simulink model "pid"  (R2018a)
settings: Solver=VariableStepAuto  StartTime=0.0  StopTime=10.0  RelTol=1e-3
settings Model: Creator=hp  LastModifiedBy=hp

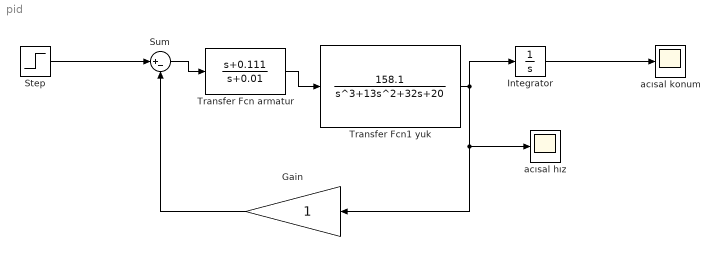
== system pid ==
  Gain : Gain
  Integrator : Integrator
  Step : Step  SampleTime=0
  Sum : Sum  Inputs=|+-
  Transfer Fcn armatur : TransferFcn  Numerator=[1 0.111]  Denominator=[1 0.01]
  Transfer Fcn1 yuk : TransferFcn  Numerator=[158.1]  Denominator=[1 13 32 20]
  acısal hız : Scope
  "acısal konum " : Scope
  wires:
  Step/1 -> Sum/1
  Sum/1 -> Transfer Fcn armatur/1
  Transfer Fcn armatur/1 -> Transfer Fcn1 yuk/1
  Transfer Fcn1 yuk/1 -> Integrator/1, Gain/1, acısal hız/1
  Integrator/1 -> "acısal konum "/1
  Gain/1 -> Sum/2
